simulink library "outp"  (Simulink 8.2)
settings: Solver=ode45  SolverMode=SingleTasking  StartTime=0.0  StopTime=10.0  RelTol=1e-3
undefined symbols (not defined in the file or in its folder): EPSILON, KOUTP_ACCSetSpeed_kph_defval, KOUTP_ACCSetSpeed_kph_maxval, KOUTP_ACCSetSpeed_kph_minval, KOUTP_ACCSetSpeed_kph_ovrdflg, KOUTP_ACCSetSpeed_kph_ovrdval, KOUTP_ACCSetSpeed_kph_srvcflg, KOUTP_ACCSetSpeed_kph_srvcval, KOUTP_ACCSetTimeGap_enum_defval, KOUTP_ACCSetTimeGap_enum_ovrdflg, KOUTP_ACCSetTimeGap_enum_ovrdval, KOUTP_ACCSetTimeGap_enum_srvcflg, KOUTP_ACCSetTimeGap_enum_srvcval, KOUTP_ACCSetTimeGapTmp_enum_defval, KOUTP_ACCSetTimeGapTmp_enum_ovrdflg, KOUTP_ACCSetTimeGapTmp_enum_ovrdval, KOUTP_ACCSetTimeGapTmp_enum_srvcflg, KOUTP_ACCSetTimeGapTmp_enum_srvcval, KOUTP_ACCWarningReq_flg_defval, KOUTP_ACCWarningReq_flg_ovrdflg, KOUTP_ACCWarningReq_flg_ovrdval, KOUTP_ACCWarningReq_flg_srvcflg, KOUTP_ACCWarningReq_flg_srvcval, KOUTP_ADAS1RollCnt_cnt_defval, KOUTP_ADAS1RollCnt_cnt_ovrdflg, KOUTP_ADAS1RollCnt_cnt_ovrdval, KOUTP_ADAS1RollCnt_cnt_srvcflg, KOUTP_ADAS1RollCnt_cnt_srvcval, KOUTP_ADAS2RollCnt_cnt_defval, KOUTP_ADAS2RollCnt_cnt_ovrdflg, KOUTP_ADAS2RollCnt_cnt_ovrdval, KOUTP_ADAS2RollCnt_cnt_srvcflg, KOUTP_ADAS2RollCnt_cnt_srvcval, KOUTP_ADAS3RollCnt_cnt_defval, KOUTP_ADAS3RollCnt_cnt_ovrdflg, KOUTP_ADAS3RollCnt_cnt_ovrdval, KOUTP_ADAS3RollCnt_cnt_srvcflg, KOUTP_ADAS3RollCnt_cnt_srvcval, KOUTP_ADASACCStatus_enum_defval, KOUTP_ADASACCStatus_enum_ovrdflg, KOUTP_ADASACCStatus_enum_ovrdval, KOUTP_ADASACCStatus_enum_srvcflg, KOUTP_ADASACCStatus_enum_srvcval, KOUTP_ADASFaultMode_enum_defval, KOUTP_ADASFaultMode_enum_ovrdflg, KOUTP_ADASFaultMode_enum_ovrdval, KOUTP_ADASFaultMode_enum_srvcflg, KOUTP_ADASFaultMode_enum_srvcval, KOUTP_ADASFunOffSoundReq_flg_defval, KOUTP_ADASFunOffSoundReq_flg_ovrdflg, KOUTP_ADASFunOffSoundReq_flg_ovrdval, KOUTP_ADASFunOffSoundReq_flg_srvcflg, KOUTP_ADASFunOffSoundReq_flg_srvcval, KOUTP_ADASFunOnSoundReq_flg_defval, KOUTP_ADASFunOnSoundReq_flg_ovrdflg, KOUTP_ADASFunOnSoundReq_flg_ovrdval, KOUTP_ADASFunOnSoundReq_flg_srvcflg, KOUTP_ADASFunOnSoundReq_flg_srvcval, KOUTP_ADASLFCStatus_enum_defval, KOUTP_ADASLFCStatus_enum_ovrdflg ... (+216)
libraries: outp x52, hcu_lib x8, simulink x3
(part 2 of 2)

== system outp/OUTP/OUTP/ADASFunOffSoundReq ==
  in : Inport
  use_default : Inport  Port=2
  KOUTP_LKAHMIStatus_enum_defval_C : Constant  Value=KOUTP_ADASFunOffSoundReq_flg_defval
  KOUTP_LKAHMIStatus_enum_ovrdflg_C : Constant  Value=KOUTP_ADASFunOffSoundReq_flg_ovrdflg
  KOUTP_LKAHMIStatus_enum_ovrdval_C : Constant  Value=KOUTP_ADASFunOffSoundReq_flg_ovrdval
  KOUTP_LKAHMIStatus_enum_srvcflg_C : Constant  Value=KOUTP_ADASFunOffSoundReq_flg_srvcflg
  KOUTP_LKAHMIStatus_enum_srvcval_C : Constant  Value=KOUTP_ADASFunOffSoundReq_flg_srvcval
  Switch1 : Switch  Criteria=u2 ~= 0  Threshold=0.5
  signal_out : outp/signal_out
  out : Outport
  wires:
  in/1 -> signal_out/1
  signal_out/1 -> Switch1/3
  use_default/1 -> Switch1/2
  Switch1/1 -> out/1
  KOUTP_LKAHMIStatus_enum_srvcflg_C/1 -> signal_out/2
  KOUTP_LKAHMIStatus_enum_srvcval_C/1 -> signal_out/3
  KOUTP_LKAHMIStatus_enum_ovrdflg_C/1 -> signal_out/4
  KOUTP_LKAHMIStatus_enum_ovrdval_C/1 -> signal_out/5
  KOUTP_LKAHMIStatus_enum_defval_C/1 -> Switch1/1

== system outp/OUTP/OUTP/ADASFunOnSoundReq ==
  in : Inport
  use_default : Inport  Port=2
  KOUTP_LKAHMIStatus_enum_defval_C : Constant  Value=KOUTP_ADASFunOnSoundReq_flg_defval
  KOUTP_LKAHMIStatus_enum_ovrdflg_C : Constant  Value=KOUTP_ADASFunOnSoundReq_flg_ovrdflg
  KOUTP_LKAHMIStatus_enum_ovrdval_C : Constant  Value=KOUTP_ADASFunOnSoundReq_flg_ovrdval
  KOUTP_LKAHMIStatus_enum_srvcflg_C : Constant  Value=KOUTP_ADASFunOnSoundReq_flg_srvcflg
  KOUTP_LKAHMIStatus_enum_srvcval_C : Constant  Value=KOUTP_ADASFunOnSoundReq_flg_srvcval
  Switch1 : Switch  Criteria=u2 ~= 0  Threshold=0.5
  signal_out : outp/signal_out
  out : Outport
  wires:
  KOUTP_LKAHMIStatus_enum_defval_C/1 -> Switch1/1
  KOUTP_LKAHMIStatus_enum_ovrdval_C/1 -> signal_out/5
  KOUTP_LKAHMIStatus_enum_ovrdflg_C/1 -> signal_out/4
  KOUTP_LKAHMIStatus_enum_srvcval_C/1 -> signal_out/3
  KOUTP_LKAHMIStatus_enum_srvcflg_C/1 -> signal_out/2
  Switch1/1 -> out/1
  use_default/1 -> Switch1/2
  signal_out/1 -> Switch1/3
  in/1 -> signal_out/1

== system outp/OUTP/OUTP/ADASLFCStatus ==
  in : Inport
  use_default : Inport  Port=2
  KOUTP_ADASLFCStatus_enum_defval_C : Constant  Value=KOUTP_ADASLFCStatus_enum_defval
  KOUTP_ADASLFCStatus_enum_ovrdflg_C : Constant  Value=KOUTP_ADASLFCStatus_enum_ovrdflg
  KOUTP_ADASLFCStatus_enum_ovrdval_C : Constant  Value=KOUTP_ADASLFCStatus_enum_ovrdval
  KOUTP_ADASLFCStatus_enum_srvcflg_C : Constant  Value=KOUTP_ADASLFCStatus_enum_srvcflg
  KOUTP_ADASLFCStatus_enum_srvcval_C : Constant  Value=KOUTP_ADASLFCStatus_enum_srvcval
  Switch1 : Switch  Criteria=u2 ~= 0  Threshold=0.5
  signal_out : outp/signal_out
  out : Outport
  wires:
  KOUTP_ADASLFCStatus_enum_defval_C/1 -> Switch1/1
  KOUTP_ADASLFCStatus_enum_ovrdval_C/1 -> signal_out/5
  KOUTP_ADASLFCStatus_enum_ovrdflg_C/1 -> signal_out/4
  KOUTP_ADASLFCStatus_enum_srvcval_C/1 -> signal_out/3
  KOUTP_ADASLFCStatus_enum_srvcflg_C/1 -> signal_out/2
  Switch1/1 -> out/1
  use_default/1 -> Switch1/2
  signal_out/1 -> Switch1/3
  in/1 -> signal_out/1

== system outp/OUTP/OUTP/ADASLKAStatus ==
  in : Inport
  use_default : Inport  Port=2
  KOUTP_ADASLKAStatus_enum_defval_C : Constant  Value=KOUTP_ADASLKAStatus_enum_defval
  KOUTP_ADASLKAStatus_enum_ovrdflg_C : Constant  Value=KOUTP_ADASLKAStatus_enum_ovrdflg
  KOUTP_ADASLKAStatus_enum_ovrdval_C : Constant  Value=KOUTP_ADASLKAStatus_enum_ovrdval
  KOUTP_ADASLKAStatus_enum_srvcflg_C : Constant  Value=KOUTP_ADASLKAStatus_enum_srvcflg
  KOUTP_ADASLKAStatus_enum_srvcval_C : Constant  Value=KOUTP_ADASLKAStatus_enum_srvcval
  Switch1 : Switch  Criteria=u2 ~= 0  Threshold=0.5
  signal_out : outp/signal_out
  out : Outport
  wires:
  in/1 -> signal_out/1
  signal_out/1 -> Switch1/3
  use_default/1 -> Switch1/2
  Switch1/1 -> out/1
  KOUTP_ADASLKAStatus_enum_srvcflg_C/1 -> signal_out/2
  KOUTP_ADASLKAStatus_enum_srvcval_C/1 -> signal_out/3
  KOUTP_ADASLKAStatus_enum_ovrdflg_C/1 -> signal_out/4
  KOUTP_ADASLKAStatus_enum_ovrdval_C/1 -> signal_out/5
  KOUTP_ADASLKAStatus_enum_defval_C/1 -> Switch1/1

== system outp/OUTP/OUTP/ADASMILReq ==
  in : Inport
  use_default : Inport  Port=2
  KOUTP_ADASMILReq_flg_defval_C : Constant  Value=KOUTP_ADASMILReq_flg_defval
  KOUTP_ADASMILReq_flg_ovrdflg_C : Constant  Value=KOUTP_ADASMILReq_flg_ovrdflg
  KOUTP_ADASMILReq_flg_ovrdval_C : Constant  Value=KOUTP_ADASMILReq_flg_ovrdval
  KOUTP_ADASMILReq_flg_srvcflg_C : Constant  Value=KOUTP_ADASMILReq_flg_srvcflg
  KOUTP_ADASMILReq_flg_srvcval_C : Constant  Value=KOUTP_ADASMILReq_flg_srvcval
  Switch1 : Switch  Criteria=u2 ~= 0  Threshold=0.5
  signal_out : outp/signal_out
  out : Outport
  wires:
  KOUTP_ADASMILReq_flg_defval_C/1 -> Switch1/1
  KOUTP_ADASMILReq_flg_ovrdval_C/1 -> signal_out/5
  KOUTP_ADASMILReq_flg_ovrdflg_C/1 -> signal_out/4
  KOUTP_ADASMILReq_flg_srvcval_C/1 -> signal_out/3
  KOUTP_ADASMILReq_flg_srvcflg_C/1 -> signal_out/2
  Switch1/1 -> out/1
  use_default/1 -> Switch1/2
  signal_out/1 -> Switch1/3
  in/1 -> signal_out/1

== system outp/OUTP/OUTP/AEBReq ==
  in : Inport
  use_default : Inport  Port=2
  KOUTP_AEBReq_flg_defval_C : Constant  Value=KOUTP_AEBReq_flg_defval
  KOUTP_AEBReq_flg_ovrdflg_C : Constant  Value=KOUTP_AEBReq_flg_ovrdflg
  KOUTP_AEBReq_flg_ovrdval_C : Constant  Value=KOUTP_AEBReq_flg_ovrdval
  KOUTP_AEBReq_flg_srvcflg_C : Constant  Value=KOUTP_AEBReq_flg_srvcflg
  KOUTP_AEBReq_flg_srvcval_C : Constant  Value=KOUTP_AEBReq_flg_srvcval
  Switch1 : Switch  Criteria=u2 ~= 0  Threshold=0.5
  signal_out : outp/signal_out
  out : Outport
  wires:
  in/1 -> signal_out/1
  signal_out/1 -> Switch1/3
  use_default/1 -> Switch1/2
  Switch1/1 -> out/1
  KOUTP_AEBReq_flg_srvcflg_C/1 -> signal_out/2
  KOUTP_AEBReq_flg_srvcval_C/1 -> signal_out/3
  KOUTP_AEBReq_flg_ovrdflg_C/1 -> signal_out/4
  KOUTP_AEBReq_flg_ovrdval_C/1 -> signal_out/5
  KOUTP_AEBReq_flg_defval_C/1 -> Switch1/1

== system outp/OUTP/OUTP/AEBReqAppl ==
  in : Inport
  use_default : Inport  Port=2
  KOUTP_AEBReqAppl_flg_defval_C : Constant  Value=KOUTP_AEBReqAppl_flg_defval
  KOUTP_AEBReqAppl_flg_ovrdflg_C : Constant  Value=KOUTP_AEBReqAppl_flg_ovrdflg
  KOUTP_AEBReqAppl_flg_ovrdval_C : Constant  Value=KOUTP_AEBReqAppl_flg_ovrdval
  KOUTP_AEBReqAppl_flg_srvcflg_C : Constant  Value=KOUTP_AEBReqAppl_flg_srvcflg
  KOUTP_AEBReqAppl_flg_srvcval_C : Constant  Value=KOUTP_AEBReqAppl_flg_srvcval
  Switch1 : Switch  Criteria=u2 ~= 0  Threshold=0.5
  signal_out : outp/signal_out
  out : Outport
  wires:
  KOUTP_AEBReqAppl_flg_defval_C/1 -> Switch1/1
  KOUTP_AEBReqAppl_flg_ovrdval_C/1 -> signal_out/5
  KOUTP_AEBReqAppl_flg_ovrdflg_C/1 -> signal_out/4
  KOUTP_AEBReqAppl_flg_srvcval_C/1 -> signal_out/3
  KOUTP_AEBReqAppl_flg_srvcflg_C/1 -> signal_out/2
  Switch1/1 -> out/1
  use_default/1 -> Switch1/2
  signal_out/1 -> Switch1/3
  in/1 -> signal_out/1

== system outp/OUTP/OUTP/AEBWarningReq ==
  in : Inport
  use_default : Inport  Port=2
  KOUTP_AEBWarningReq_flg_defval_C : Constant  Value=KOUTP_AEBWarningReq_flg_defval
  KOUTP_AEBWarningReq_flg_ovrdflg_C : Constant  Value=KOUTP_AEBWarningReq_flg_ovrdflg
  KOUTP_AEBWarningReq_flg_ovrdval_C : Constant  Value=KOUTP_AEBWarningReq_flg_ovrdval
  KOUTP_AEBWarningReq_flg_srvcflg_C : Constant  Value=KOUTP_AEBWarningReq_flg_srvcflg
  KOUTP_AEBWarningReq_flg_srvcval_C : Constant  Value=KOUTP_AEBWarningReq_flg_srvcval
  Switch1 : Switch  Criteria=u2 ~= 0  Threshold=0.5
  signal_out : outp/signal_out
  out : Outport
  wires:
  KOUTP_AEBWarningReq_flg_defval_C/1 -> Switch1/1
  KOUTP_AEBWarningReq_flg_ovrdval_C/1 -> signal_out/5
  KOUTP_AEBWarningReq_flg_ovrdflg_C/1 -> signal_out/4
  KOUTP_AEBWarningReq_flg_srvcval_C/1 -> signal_out/3
  KOUTP_AEBWarningReq_flg_srvcflg_C/1 -> signal_out/2
  Switch1/1 -> out/1
  use_default/1 -> Switch1/2
  signal_out/1 -> Switch1/3
  in/1 -> signal_out/1

== system outp/OUTP/OUTP/BrakeHapticReq ==
  in : Inport
  use_default : Inport  Port=2
  KOUTP_BrakeHapticReq_flg_defval_C : Constant  Value=KOUTP_BrakeHapticReq_flg_defval
  KOUTP_BrakeHapticReq_flg_ovrdflg_C : Constant  Value=KOUTP_BrakeHapticReq_flg_ovrdflg
  KOUTP_BrakeHapticReq_flg_ovrdval_C : Constant  Value=KOUTP_BrakeHapticReq_flg_ovrdval
  KOUTP_BrakeHapticReq_flg_srvcflg_C : Constant  Value=KOUTP_BrakeHapticReq_flg_srvcflg
  KOUTP_BrakeHapticReq_flg_srvcval_C : Constant  Value=KOUTP_BrakeHapticReq_flg_srvcval
  Switch1 : Switch  Criteria=u2 ~= 0  Threshold=0.5
  signal_out : outp/signal_out
  out : Outport
  wires:
  KOUTP_BrakeHapticReq_flg_defval_C/1 -> Switch1/1
  KOUTP_BrakeHapticReq_flg_ovrdval_C/1 -> signal_out/5
  KOUTP_BrakeHapticReq_flg_ovrdflg_C/1 -> signal_out/4
  KOUTP_BrakeHapticReq_flg_srvcval_C/1 -> signal_out/3
  KOUTP_BrakeHapticReq_flg_srvcflg_C/1 -> signal_out/2
  Switch1/1 -> out/1
  use_default/1 -> Switch1/2
  signal_out/1 -> Switch1/3
  in/1 -> signal_out/1

== system outp/OUTP/OUTP/BrakePrefillReq ==
  in : Inport
  use_default : Inport  Port=2
  KOUTP_BrakePrefillReq_flg_defval_C : Constant  Value=KOUTP_BrakePrefillReq_flg_defval
  KOUTP_BrakePrefillReq_flg_ovrdflg_C : Constant  Value=KOUTP_BrakePrefillReq_flg_ovrdflg
  KOUTP_BrakePrefillReq_flg_ovrdval_C : Constant  Value=KOUTP_BrakePrefillReq_flg_ovrdval
  KOUTP_BrakePrefillReq_flg_srvcflg_C : Constant  Value=KOUTP_BrakePrefillReq_flg_srvcflg
  KOUTP_BrakePrefillReq_flg_srvcval_C : Constant  Value=KOUTP_BrakePrefillReq_flg_srvcval
  Switch1 : Switch  Criteria=u2 ~= 0  Threshold=0.5
  signal_out : outp/signal_out
  out : Outport
  wires:
  in/1 -> signal_out/1
  signal_out/1 -> Switch1/3
  use_default/1 -> Switch1/2
  Switch1/1 -> out/1
  KOUTP_BrakePrefillReq_flg_srvcflg_C/1 -> signal_out/2
  KOUTP_BrakePrefillReq_flg_srvcval_C/1 -> signal_out/3
  KOUTP_BrakePrefillReq_flg_ovrdflg_C/1 -> signal_out/4
  KOUTP_BrakePrefillReq_flg_ovrdval_C/1 -> signal_out/5
  KOUTP_BrakePrefillReq_flg_defval_C/1 -> Switch1/1

== system outp/OUTP/OUTP/BrakePrefillReqAppl ==
  in : Inport
  use_default : Inport  Port=2
  KOUTP_BrakePrefillReqAppl_flg_defval_C : Constant  Value=KOUTP_BrakePrefillReqAppl_flg_defval
  KOUTP_BrakePrefillReqAppl_flg_ovrdflg_C : Constant  Value=KOUTP_BrakePrefillReqAppl_flg_ovrdflg
  KOUTP_BrakePrefillReqAppl_flg_ovrdval_C : Constant  Value=KOUTP_BrakePrefillReqAppl_flg_ovrdval
  KOUTP_BrakePrefillReqAppl_flg_srvcflg_C : Constant  Value=KOUTP_BrakePrefillReqAppl_flg_srvcflg
  KOUTP_BrakePrefillReqAppl_flg_srvcval_C : Constant  Value=KOUTP_BrakePrefillReqAppl_flg_srvcval
  Switch1 : Switch  Criteria=u2 ~= 0  Threshold=0.5
  signal_out : outp/signal_out
  out : Outport
  wires:
  KOUTP_BrakePrefillReqAppl_flg_defval_C/1 -> Switch1/1
  KOUTP_BrakePrefillReqAppl_flg_ovrdval_C/1 -> signal_out/5
  KOUTP_BrakePrefillReqAppl_flg_ovrdflg_C/1 -> signal_out/4
  KOUTP_BrakePrefillReqAppl_flg_srvcval_C/1 -> signal_out/3
  KOUTP_BrakePrefillReqAppl_flg_srvcflg_C/1 -> signal_out/2
  Switch1/1 -> out/1
  use_default/1 -> Switch1/2
  signal_out/1 -> Switch1/3
  in/1 -> signal_out/1

== system outp/OUTP/OUTP/DecReq ==
  in : Inport
  use_default : Inport  Port=2
  KOUTP_DecReq_mps2_defval_C : Constant  Value=KOUTP_DecReq_mps2_defval
  KOUTP_DecReq_mps2_ovrdflg_C : Constant  Value=KOUTP_DecReq_mps2_ovrdflg
  KOUTP_DecReq_mps2_ovrdval_C : Constant  Value=KOUTP_DecReq_mps2_ovrdval
  KOUTP_DecReq_mps2_srvcflg_C : Constant  Value=KOUTP_DecReq_mps2_srvcflg
  KOUTP_DecReq_mps2_srvcval_C : Constant  Value=KOUTP_DecReq_mps2_srvcval
  Switch1 : Switch  Criteria=u2 ~= 0  Threshold=0.5
  signal_out : outp/signal_out
  out : Outport
  wires:
  in/1 -> signal_out/1
  signal_out/1 -> Switch1/3
  use_default/1 -> Switch1/2
  Switch1/1 -> out/1
  KOUTP_DecReq_mps2_srvcflg_C/1 -> signal_out/2
  KOUTP_DecReq_mps2_srvcval_C/1 -> signal_out/3
  KOUTP_DecReq_mps2_ovrdflg_C/1 -> signal_out/4
  KOUTP_DecReq_mps2_ovrdval_C/1 -> signal_out/5
  KOUTP_DecReq_mps2_defval_C/1 -> Switch1/1

== system outp/OUTP/OUTP/DecReqAppl ==
  in : Inport
  use_default : Inport  Port=2
  KOUTP_DecReqAppl_flg_defval_C : Constant  Value=KOUTP_DecReqAppl_flg_defval
  KOUTP_DecReqAppl_flg_ovrdflg_C : Constant  Value=KOUTP_DecReqAppl_flg_ovrdflg
  KOUTP_DecReqAppl_flg_ovrdval_C : Constant  Value=KOUTP_DecReqAppl_flg_ovrdval
  KOUTP_DecReqAppl_flg_srvcflg_C : Constant  Value=KOUTP_DecReqAppl_flg_srvcflg
  KOUTP_DecReqAppl_flg_srvcval_C : Constant  Value=KOUTP_DecReqAppl_flg_srvcval
  Switch1 : Switch  Criteria=u2 ~= 0  Threshold=0.5
  signal_out : outp/signal_out
  out : Outport
  wires:
  KOUTP_DecReqAppl_flg_defval_C/1 -> Switch1/1
  KOUTP_DecReqAppl_flg_ovrdval_C/1 -> signal_out/5
  KOUTP_DecReqAppl_flg_ovrdflg_C/1 -> signal_out/4
  KOUTP_DecReqAppl_flg_srvcval_C/1 -> signal_out/3
  KOUTP_DecReqAppl_flg_srvcflg_C/1 -> signal_out/2
  Switch1/1 -> out/1
  use_default/1 -> Switch1/2
  signal_out/1 -> Switch1/3
  in/1 -> signal_out/1

== system outp/OUTP/OUTP/EPSModeReq ==
  in : Inport
  use_default : Inport  Port=2
  KOUTP_EPSModeReq_enum_defval_C : Constant  Value=KOUTP_EPSModeReq_enum_defval
  KOUTP_EPSModeReq_enum_ovrdflg_C : Constant  Value=KOUTP_EPSModeReq_enum_ovrdflg
  KOUTP_EPSModeReq_enum_ovrdval_C : Constant  Value=KOUTP_EPSModeReq_enum_ovrdval
  KOUTP_EPSModeReq_enum_srvcflg_C : Constant  Value=KOUTP_EPSModeReq_enum_srvcflg
  KOUTP_EPSModeReq_enum_srvcval_C : Constant  Value=KOUTP_EPSModeReq_enum_srvcval
  Switch1 : Switch  Criteria=u2 ~= 0  Threshold=0.5
  signal_out : outp/signal_out
  out : Outport
  wires:
  KOUTP_EPSModeReq_enum_defval_C/1 -> Switch1/1
  KOUTP_EPSModeReq_enum_ovrdval_C/1 -> signal_out/5
  KOUTP_EPSModeReq_enum_ovrdflg_C/1 -> signal_out/4
  KOUTP_EPSModeReq_enum_srvcval_C/1 -> signal_out/3
  KOUTP_EPSModeReq_enum_srvcflg_C/1 -> signal_out/2
  Switch1/1 -> out/1
  use_default/1 -> Switch1/2
  signal_out/1 -> Switch1/3
  in/1 -> signal_out/1

== system outp/OUTP/OUTP/FCWWarningReq ==
  in : Inport
  use_default : Inport  Port=2
  KOUTP_FCWWarningReq_flg_defval_C : Constant  Value=KOUTP_FCWWarningReq_flg_defval
  KOUTP_FCWWarningReq_flg_ovrdflg_C : Constant  Value=KOUTP_FCWWarningReq_flg_ovrdflg
  KOUTP_FCWWarningReq_flg_ovrdval_C : Constant  Value=KOUTP_FCWWarningReq_flg_ovrdval
  KOUTP_FCWWarningReq_flg_srvcflg_C : Constant  Value=KOUTP_FCWWarningReq_flg_srvcflg
  KOUTP_FCWWarningReq_flg_srvcval_C : Constant  Value=KOUTP_FCWWarningReq_flg_srvcval
  Switch1 : Switch  Criteria=u2 ~= 0  Threshold=0.5
  signal_out : outp/signal_out
  out : Outport
  wires:
  KOUTP_FCWWarningReq_flg_defval_C/1 -> Switch1/1
  KOUTP_FCWWarningReq_flg_ovrdval_C/1 -> signal_out/5
  KOUTP_FCWWarningReq_flg_ovrdflg_C/1 -> signal_out/4
  KOUTP_FCWWarningReq_flg_srvcval_C/1 -> signal_out/3
  KOUTP_FCWWarningReq_flg_srvcflg_C/1 -> signal_out/2
  Switch1/1 -> out/1
  use_default/1 -> Switch1/2
  signal_out/1 -> Switch1/3
  in/1 -> signal_out/1

== system outp/OUTP/OUTP/FaultWarningReq ==
  in : Inport
  use_default : Inport  Port=2
  KOUTP_FaultWarningReq_flg_defval_C : Constant  Value=KOUTP_FaultWarningReq_flg_defval
  KOUTP_FaultWarningReq_flg_ovrdflg_C : Constant  Value=KOUTP_FaultWarningReq_flg_ovrdflg
  KOUTP_FaultWarningReq_flg_ovrdval_C : Constant  Value=KOUTP_FaultWarningReq_flg_ovrdval
  KOUTP_FaultWarningReq_flg_srvcflg_C : Constant  Value=KOUTP_FaultWarningReq_flg_srvcflg
  KOUTP_FaultWarningReq_flg_srvcval_C : Constant  Value=KOUTP_FaultWarningReq_flg_srvcval
  Switch1 : Switch  Criteria=u2 ~= 0  Threshold=0.5
  signal_out : outp/signal_out
  out : Outport
  wires:
  KOUTP_FaultWarningReq_flg_defval_C/1 -> Switch1/1
  KOUTP_FaultWarningReq_flg_ovrdval_C/1 -> signal_out/5
  KOUTP_FaultWarningReq_flg_ovrdflg_C/1 -> signal_out/4
  KOUTP_FaultWarningReq_flg_srvcval_C/1 -> signal_out/3
  KOUTP_FaultWarningReq_flg_srvcflg_C/1 -> signal_out/2
  Switch1/1 -> out/1
  use_default/1 -> Switch1/2
  signal_out/1 -> Switch1/3
  in/1 -> signal_out/1

== system outp/OUTP/OUTP/ForceIdle ==
  in : Inport
  use_default : Inport  Port=2
  KOUTP_ForceIdle_flg_defval_C : Constant  Value=KOUTP_ForceIdle_flg_defval
  KOUTP_ForceIdle_flg_ovrdflg_C : Constant  Value=KOUTP_ForceIdle_flg_ovrdflg
  KOUTP_ForceIdle_flg_ovrdval_C : Constant  Value=KOUTP_ForceIdle_flg_ovrdval
  KOUTP_ForceIdle_flg_srvcflg_C : Constant  Value=KOUTP_ForceIdle_flg_srvcflg
  KOUTP_ForceIdle_flg_srvcval_C : Constant  Value=KOUTP_ForceIdle_flg_srvcval
  Switch1 : Switch  Criteria=u2 ~= 0  Threshold=0.5
  signal_out : outp/signal_out
  out : Outport
  wires:
  KOUTP_ForceIdle_flg_defval_C/1 -> Switch1/1
  KOUTP_ForceIdle_flg_ovrdval_C/1 -> signal_out/5
  KOUTP_ForceIdle_flg_ovrdflg_C/1 -> signal_out/4
  KOUTP_ForceIdle_flg_srvcval_C/1 -> signal_out/3
  KOUTP_ForceIdle_flg_srvcflg_C/1 -> signal_out/2
  Switch1/1 -> out/1
  use_default/1 -> Switch1/2
  signal_out/1 -> Switch1/3
  in/1 -> signal_out/1

== system outp/OUTP/OUTP/ForceIdleAppl ==
  in : Inport
  use_default : Inport  Port=2
  KOUTP_ForceIdleAppl_flg_defval_C : Constant  Value=KOUTP_ForceIdleAppl_flg_defval
  KOUTP_ForceIdleAppl_flg_ovrdflg_C : Constant  Value=KOUTP_ForceIdleAppl_flg_ovrdflg
  KOUTP_ForceIdleAppl_flg_ovrdval_C : Constant  Value=KOUTP_ForceIdleAppl_flg_ovrdval
  KOUTP_ForceIdleAppl_flg_srvcflg_C : Constant  Value=KOUTP_ForceIdleAppl_flg_srvcflg
  KOUTP_ForceIdleAppl_flg_srvcval_C : Constant  Value=KOUTP_ForceIdleAppl_flg_srvcval
  Switch1 : Switch  Criteria=u2 ~= 0  Threshold=0.5
  signal_out : outp/signal_out
  out : Outport
  wires:
  in/1 -> signal_out/1
  signal_out/1 -> Switch1/3
  use_default/1 -> Switch1/2
  Switch1/1 -> out/1
  KOUTP_ForceIdleAppl_flg_srvcflg_C/1 -> signal_out/2
  KOUTP_ForceIdleAppl_flg_srvcval_C/1 -> signal_out/3
  KOUTP_ForceIdleAppl_flg_ovrdflg_C/1 -> signal_out/4
  KOUTP_ForceIdleAppl_flg_ovrdval_C/1 -> signal_out/5
  KOUTP_ForceIdleAppl_flg_defval_C/1 -> Switch1/1

== system outp/OUTP/OUTP/ForceLowBeam ==
  in : Inport
  use_default : Inport  Port=2
  KOUTP_ADASMILReq_flg_defval_C : Constant  Value=KOUTP_ForceLowBeam_flg_defval
  KOUTP_ADASMILReq_flg_ovrdflg_C : Constant  Value=KOUTP_ForceLowBeam_flg_ovrdflg
  KOUTP_ADASMILReq_flg_ovrdval_C : Constant  Value=KOUTP_ForceLowBeam_flg_ovrdval
  KOUTP_ADASMILReq_flg_srvcflg_C : Constant  Value=KOUTP_ForceLowBeam_flg_srvcflg
  KOUTP_ADASMILReq_flg_srvcval_C : Constant  Value=KOUTP_ForceLowBeam_flg_srvcval
  Switch1 : Switch  Criteria=u2 ~= 0  Threshold=0.5
  signal_out : outp/signal_out
  out : Outport
  wires:
  in/1 -> signal_out/1
  signal_out/1 -> Switch1/3
  use_default/1 -> Switch1/2
  Switch1/1 -> out/1
  KOUTP_ADASMILReq_flg_srvcflg_C/1 -> signal_out/2
  KOUTP_ADASMILReq_flg_srvcval_C/1 -> signal_out/3
  KOUTP_ADASMILReq_flg_ovrdflg_C/1 -> signal_out/4
  KOUTP_ADASMILReq_flg_ovrdval_C/1 -> signal_out/5
  KOUTP_ADASMILReq_flg_defval_C/1 -> Switch1/1

== system outp/OUTP/OUTP/GearPosnReq ==
  in : Inport
  use_default : Inport  Port=2
  KOUTP_GearPosnReq_enum_defval_C : Constant  Value=KOUTP_GearPosnReq_enum_defval
  KOUTP_GearPosnReq_enum_ovrdflg_C : Constant  Value=KOUTP_GearPosnReq_enum_ovrdflg
  KOUTP_GearPosnReq_enum_ovrdval_C : Constant  Value=KOUTP_GearPosnReq_enum_ovrdval
  KOUTP_GearPosnReq_enum_srvcflg_C : Constant  Value=KOUTP_GearPosnReq_enum_srvcflg
  KOUTP_GearPosnReq_enum_srvcval_C : Constant  Value=KOUTP_GearPosnReq_enum_srvcval
  Switch1 : Switch  Criteria=u2 ~= 0  Threshold=0.5
  signal_out : outp/signal_out
  out : Outport
  wires:
  KOUTP_GearPosnReq_enum_defval_C/1 -> Switch1/1
  KOUTP_GearPosnReq_enum_ovrdval_C/1 -> signal_out/5
  KOUTP_GearPosnReq_enum_ovrdflg_C/1 -> signal_out/4
  KOUTP_GearPosnReq_enum_srvcval_C/1 -> signal_out/3
  KOUTP_GearPosnReq_enum_srvcflg_C/1 -> signal_out/2
  Switch1/1 -> out/1
  use_default/1 -> Switch1/2
  signal_out/1 -> Switch1/3
  in/1 -> signal_out/1

== system outp/OUTP/OUTP/GearPosnReqAppl ==
  in : Inport
  use_default : Inport  Port=2
  KOUTP_GearPosnReqAppl_flg_defval_C : Constant  Value=KOUTP_GearPosnReqAppl_flg_defval
  KOUTP_GearPosnReqAppl_flg_ovrdflg_C : Constant  Value=KOUTP_GearPosnReqAppl_flg_ovrdflg
  KOUTP_GearPosnReqAppl_flg_ovrdval_C : Constant  Value=KOUTP_GearPosnReqAppl_flg_ovrdval
  KOUTP_GearPosnReqAppl_flg_srvcflg_C : Constant  Value=KOUTP_GearPosnReqAppl_flg_srvcflg
  KOUTP_GearPosnReqAppl_flg_srvcval_C : Constant  Value=KOUTP_GearPosnReqAppl_flg_srvcval
  Switch1 : Switch  Criteria=u2 ~= 0  Threshold=0.5
  signal_out : outp/signal_out
  out : Outport
  wires:
  in/1 -> signal_out/1
  signal_out/1 -> Switch1/3
  use_default/1 -> Switch1/2
  Switch1/1 -> out/1
  KOUTP_GearPosnReqAppl_flg_srvcflg_C/1 -> signal_out/2
  KOUTP_GearPosnReqAppl_flg_srvcval_C/1 -> signal_out/3
  KOUTP_GearPosnReqAppl_flg_ovrdflg_C/1 -> signal_out/4
  KOUTP_GearPosnReqAppl_flg_ovrdval_C/1 -> signal_out/5
  KOUTP_GearPosnReqAppl_flg_defval_C/1 -> Switch1/1

== system outp/OUTP/OUTP/HazardWarningReq ==
  in : Inport
  use_default : Inport  Port=2
  KOUTP_HazardWarningReq_flg_defval_C : Constant  Value=KOUTP_HazardWarningReq_flg_defval
  KOUTP_HazardWarningReq_flg_ovrdflg_C : Constant  Value=KOUTP_HazardWarningReq_flg_ovrdflg
  KOUTP_HazardWarningReq_flg_ovrdval_C : Constant  Value=KOUTP_HazardWarningReq_flg_ovrdval
  KOUTP_HazardWarningReq_flg_srvcflg_C : Constant  Value=KOUTP_HazardWarningReq_flg_srvcflg
  KOUTP_HazardWarningReq_flg_srvcval_C : Constant  Value=KOUTP_HazardWarningReq_flg_srvcval
  Switch1 : Switch  Criteria=u2 ~= 0  Threshold=0.5
  signal_out : outp/signal_out
  out : Outport
  wires:
  in/1 -> signal_out/1
  signal_out/1 -> Switch1/3
  use_default/1 -> Switch1/2
  Switch1/1 -> out/1
  KOUTP_HazardWarningReq_flg_srvcflg_C/1 -> signal_out/2
  KOUTP_HazardWarningReq_flg_srvcval_C/1 -> signal_out/3
  KOUTP_HazardWarningReq_flg_ovrdflg_C/1 -> signal_out/4
  KOUTP_HazardWarningReq_flg_ovrdval_C/1 -> signal_out/5
  KOUTP_HazardWarningReq_flg_defval_C/1 -> Switch1/1

== system outp/OUTP/OUTP/IGSAWarningReq ==
  in : Inport
  use_default : Inport  Port=2
  KOUTP_IGSAWarningReq_flg_defval_C : Constant  Value=KOUTP_IGSAWarningReq_flg_defval
  KOUTP_IGSAWarningReq_flg_ovrdflg_C : Constant  Value=KOUTP_IGSAWarningReq_flg_ovrdflg
  KOUTP_IGSAWarningReq_flg_ovrdval_C : Constant  Value=KOUTP_IGSAWarningReq_flg_ovrdval
  KOUTP_IGSAWarningReq_flg_srvcflg_C : Constant  Value=KOUTP_IGSAWarningReq_flg_srvcflg
  KOUTP_IGSAWarningReq_flg_srvcval_C : Constant  Value=KOUTP_IGSAWarningReq_flg_srvcval
  Switch1 : Switch  Criteria=u2 ~= 0  Threshold=0.5
  signal_out : outp/signal_out
  out : Outport
  wires:
  in/1 -> signal_out/1
  signal_out/1 -> Switch1/3
  use_default/1 -> Switch1/2
  Switch1/1 -> out/1
  KOUTP_IGSAWarningReq_flg_srvcflg_C/1 -> signal_out/2
  KOUTP_IGSAWarningReq_flg_srvcval_C/1 -> signal_out/3
  KOUTP_IGSAWarningReq_flg_ovrdflg_C/1 -> signal_out/4
  KOUTP_IGSAWarningReq_flg_ovrdval_C/1 -> signal_out/5
  KOUTP_IGSAWarningReq_flg_defval_C/1 -> Switch1/1

== system outp/OUTP/OUTP/LFCHMIStatus ==
  in : Inport
  use_default : Inport  Port=2
  KOUTP_LFCHMIStatus_enum_defval_C : Constant  Value=KOUTP_LFCHMIStatus_enum_defval
  KOUTP_LFCHMIStatus_enum_ovrdflg_C : Constant  Value=KOUTP_LFCHMIStatus_enum_ovrdflg
  KOUTP_LFCHMIStatus_enum_ovrdval_C : Constant  Value=KOUTP_LFCHMIStatus_enum_ovrdval
  KOUTP_LFCHMIStatus_enum_srvcflg_C : Constant  Value=KOUTP_LFCHMIStatus_enum_srvcflg
  KOUTP_LFCHMIStatus_enum_srvcval_C : Constant  Value=KOUTP_LFCHMIStatus_enum_srvcval
  Switch1 : Switch  Criteria=u2 ~= 0  Threshold=0.5
  signal_out : outp/signal_out
  out : Outport
  wires:
  in/1 -> signal_out/1
  signal_out/1 -> Switch1/3
  use_default/1 -> Switch1/2
  Switch1/1 -> out/1
  KOUTP_LFCHMIStatus_enum_srvcflg_C/1 -> signal_out/2
  KOUTP_LFCHMIStatus_enum_srvcval_C/1 -> signal_out/3
  KOUTP_LFCHMIStatus_enum_ovrdflg_C/1 -> signal_out/4
  KOUTP_LFCHMIStatus_enum_ovrdval_C/1 -> signal_out/5
  KOUTP_LFCHMIStatus_enum_defval_C/1 -> Switch1/1

== system outp/OUTP/OUTP/LFCTransGain ==
  in : Inport
  use_default : Inport  Port=2
  KOUTP_LFCTransGain_rat_defval_C : Constant  Value=KOUTP_LFCTransGain_rat_defval
  KOUTP_LFCTransGain_rat_ovrdflg_C : Constant  Value=KOUTP_LFCTransGain_rat_ovrdflg
  KOUTP_LFCTransGain_rat_ovrdval_C : Constant  Value=KOUTP_LFCTransGain_rat_ovrdval
  KOUTP_LFCTransGain_rat_srvcflg_C : Constant  Value=KOUTP_LFCTransGain_rat_srvcflg
  KOUTP_LFCTransGain_rat_srvcval_C : Constant  Value=KOUTP_LFCTransGain_rat_srvcval
  Switch1 : Switch  Criteria=u2 ~= 0  Threshold=0.5
  signal_out : outp/signal_out
  out : Outport
  wires:
  in/1 -> signal_out/1
  signal_out/1 -> Switch1/3
  use_default/1 -> Switch1/2
  Switch1/1 -> out/1
  KOUTP_LFCTransGain_rat_srvcflg_C/1 -> signal_out/2
  KOUTP_LFCTransGain_rat_srvcval_C/1 -> signal_out/3
  KOUTP_LFCTransGain_rat_ovrdflg_C/1 -> signal_out/4
  KOUTP_LFCTransGain_rat_ovrdval_C/1 -> signal_out/5
  KOUTP_LFCTransGain_rat_defval_C/1 -> Switch1/1

== system outp/OUTP/OUTP/LFCTransGainAppl ==
  in : Inport
  use_default : Inport  Port=2
  KOUTP_LFCTransGainAppl_flg_defval_C : Constant  Value=KOUTP_LFCTransGainAppl_flg_defval
  KOUTP_LFCTransGainAppl_flg_ovrdflg_C : Constant  Value=KOUTP_LFCTransGainAppl_flg_ovrdflg
  KOUTP_LFCTransGainAppl_flg_ovrdval_C : Constant  Value=KOUTP_LFCTransGainAppl_flg_ovrdval
  KOUTP_LFCTransGainAppl_flg_srvcflg_C : Constant  Value=KOUTP_LFCTransGainAppl_flg_srvcflg
  KOUTP_LFCTransGainAppl_flg_srvcval_C : Constant  Value=KOUTP_LFCTransGainAppl_flg_srvcval
  Switch1 : Switch  Criteria=u2 ~= 0  Threshold=0.5
  signal_out : outp/signal_out
  out : Outport
  wires:
  in/1 -> signal_out/1
  signal_out/1 -> Switch1/3
  use_default/1 -> Switch1/2
  Switch1/1 -> out/1
  KOUTP_LFCTransGainAppl_flg_srvcflg_C/1 -> signal_out/2
  KOUTP_LFCTransGainAppl_flg_srvcval_C/1 -> signal_out/3
  KOUTP_LFCTransGainAppl_flg_ovrdflg_C/1 -> signal_out/4
  KOUTP_LFCTransGainAppl_flg_ovrdval_C/1 -> signal_out/5
  KOUTP_LFCTransGainAppl_flg_defval_C/1 -> Switch1/1

== system outp/OUTP/OUTP/LFCWarningReq ==
  in : Inport
  use_default : Inport  Port=2
  KOUTP_LKAHMIStatus_enum_defval_C : Constant  Value=KOUTP_LFCWarningReq_flg_defval
  KOUTP_LKAHMIStatus_enum_ovrdflg_C : Constant  Value=KOUTP_LFCWarningReq_flg_ovrdflg
  KOUTP_LKAHMIStatus_enum_ovrdval_C : Constant  Value=KOUTP_LFCWarningReq_flg_ovrdval
  KOUTP_LKAHMIStatus_enum_srvcflg_C : Constant  Value=KOUTP_LFCWarningReq_flg_srvcflg
  KOUTP_LKAHMIStatus_enum_srvcval_C : Constant  Value=KOUTP_LFCWarningReq_flg_srvcval
  Switch1 : Switch  Criteria=u2 ~= 0  Threshold=0.5
  signal_out : outp/signal_out
  out : Outport
  wires:
  in/1 -> signal_out/1
  signal_out/1 -> Switch1/3
  use_default/1 -> Switch1/2
  Switch1/1 -> out/1
  KOUTP_LKAHMIStatus_enum_srvcflg_C/1 -> signal_out/2
  KOUTP_LKAHMIStatus_enum_srvcval_C/1 -> signal_out/3
  KOUTP_LKAHMIStatus_enum_ovrdflg_C/1 -> signal_out/4
  KOUTP_LKAHMIStatus_enum_ovrdval_C/1 -> signal_out/5
  KOUTP_LKAHMIStatus_enum_defval_C/1 -> Switch1/1

== system outp/OUTP/OUTP/LKAHMIStatus ==
  in : Inport
  use_default : Inport  Port=2
  KOUTP_LKAHMIStatus_enum_defval_C : Constant  Value=KOUTP_LKAHMIStatus_enum_defval
  KOUTP_LKAHMIStatus_enum_ovrdflg_C : Constant  Value=KOUTP_LKAHMIStatus_enum_ovrdflg
  KOUTP_LKAHMIStatus_enum_ovrdval_C : Constant  Value=KOUTP_LKAHMIStatus_enum_ovrdval
  KOUTP_LKAHMIStatus_enum_srvcflg_C : Constant  Value=KOUTP_LKAHMIStatus_enum_srvcflg
  KOUTP_LKAHMIStatus_enum_srvcval_C : Constant  Value=KOUTP_LKAHMIStatus_enum_srvcval
  Switch1 : Switch  Criteria=u2 ~= 0  Threshold=0.5
  signal_out : outp/signal_out
  out : Outport
  wires:
  KOUTP_LKAHMIStatus_enum_defval_C/1 -> Switch1/1
  KOUTP_LKAHMIStatus_enum_ovrdval_C/1 -> signal_out/5
  KOUTP_LKAHMIStatus_enum_ovrdflg_C/1 -> signal_out/4
  KOUTP_LKAHMIStatus_enum_srvcval_C/1 -> signal_out/3
  KOUTP_LKAHMIStatus_enum_srvcflg_C/1 -> signal_out/2
  Switch1/1 -> out/1
  use_default/1 -> Switch1/2
  signal_out/1 -> Switch1/3
  in/1 -> signal_out/1

== system outp/OUTP/OUTP/LeftLaneLampMode ==
  in : Inport
  use_default : Inport  Port=2
  KOUTP_LeftLaneLampMode_enum_defval_C : Constant  Value=KOUTP_LeftLaneLampMode_enum_defval
  KOUTP_LeftLaneLampMode_enum_ovrdflg_C : Constant  Value=KOUTP_LeftLaneLampMode_enum_ovrdflg
  KOUTP_LeftLaneLampMode_enum_ovrdval_C : Constant  Value=KOUTP_LeftLaneLampMode_enum_ovrdval
  KOUTP_LeftLaneLampMode_enum_srvcflg_C : Constant  Value=KOUTP_LeftLaneLampMode_enum_srvcflg
  KOUTP_LeftLaneLampMode_enum_srvcval_C : Constant  Value=KOUTP_LeftLaneLampMode_enum_srvcval
  Switch1 : Switch  Criteria=u2 ~= 0  Threshold=0.5
  signal_out : outp/signal_out
  out : Outport
  wires:
  in/1 -> signal_out/1
  signal_out/1 -> Switch1/3
  use_default/1 -> Switch1/2
  Switch1/1 -> out/1
  KOUTP_LeftLaneLampMode_enum_srvcflg_C/1 -> signal_out/2
  KOUTP_LeftLaneLampMode_enum_srvcval_C/1 -> signal_out/3
  KOUTP_LeftLaneLampMode_enum_ovrdflg_C/1 -> signal_out/4
  KOUTP_LeftLaneLampMode_enum_ovrdval_C/1 -> signal_out/5
  KOUTP_LeftLaneLampMode_enum_defval_C/1 -> Switch1/1

== system outp/OUTP/OUTP/NumberOfTargets ==
  in : Inport
  use_default : Inport  Port=2
  KOUTP_LKAHMIStatus_enum_defval_C : Constant  Value=KOUTP_NumberOfTargets_num_defval
  KOUTP_LKAHMIStatus_enum_ovrdflg_C : Constant  Value=KOUTP_NumberOfTargets_num_ovrdflg
  KOUTP_LKAHMIStatus_enum_ovrdval_C : Constant  Value=KOUTP_NumberOfTargets_num_ovrdval
  KOUTP_LKAHMIStatus_enum_srvcflg_C : Constant  Value=KOUTP_NumberOfTargets_num_srvcflg
  KOUTP_LKAHMIStatus_enum_srvcval_C : Constant  Value=KOUTP_NumberOfTargets_num_srvcval
  Switch1 : Switch  Criteria=u2 ~= 0  Threshold=0.5
  signal_out : outp/signal_out
  out : Outport
  wires:
  in/1 -> signal_out/1
  signal_out/1 -> Switch1/3
  use_default/1 -> Switch1/2
  Switch1/1 -> out/1
  KOUTP_LKAHMIStatus_enum_srvcflg_C/1 -> signal_out/2
  KOUTP_LKAHMIStatus_enum_srvcval_C/1 -> signal_out/3
  KOUTP_LKAHMIStatus_enum_ovrdflg_C/1 -> signal_out/4
  KOUTP_LKAHMIStatus_enum_ovrdval_C/1 -> signal_out/5
  KOUTP_LKAHMIStatus_enum_defval_C/1 -> Switch1/1

== system outp/OUTP/OUTP/PTTqReq ==
  in : Inport
  use_default : Inport  Port=2
  KOUTP_PTTqReq_Nm_defval_C : Constant  Value=KOUTP_PTTqReq_Nm_defval
  KOUTP_PTTqReq_Nm_ovrdflg_C : Constant  Value=KOUTP_PTTqReq_Nm_ovrdflg
  KOUTP_PTTqReq_Nm_ovrdval_C : Constant  Value=KOUTP_PTTqReq_Nm_ovrdval
  KOUTP_PTTqReq_Nm_srvcflg_C : Constant  Value=KOUTP_PTTqReq_Nm_srvcflg
  KOUTP_PTTqReq_Nm_srvcval_C : Constant  Value=KOUTP_PTTqReq_Nm_srvcval
  Switch1 : Switch  Criteria=u2 ~= 0  Threshold=0.5
  signal_out : outp/signal_out
  out : Outport
  wires:
  KOUTP_PTTqReq_Nm_defval_C/1 -> Switch1/1
  KOUTP_PTTqReq_Nm_ovrdval_C/1 -> signal_out/5
  KOUTP_PTTqReq_Nm_ovrdflg_C/1 -> signal_out/4
  KOUTP_PTTqReq_Nm_srvcval_C/1 -> signal_out/3
  KOUTP_PTTqReq_Nm_srvcflg_C/1 -> signal_out/2
  Switch1/1 -> out/1
  use_default/1 -> Switch1/2
  signal_out/1 -> Switch1/3
  in/1 -> signal_out/1

== system outp/OUTP/OUTP/PTTqReqAppl ==
  in : Inport
  use_default : Inport  Port=2
  KOUTP_PTTqReqAppl_flg_defval_C : Constant  Value=KOUTP_PTTqReqAppl_flg_defval
  KOUTP_PTTqReqAppl_flg_ovrdflg_C : Constant  Value=KOUTP_PTTqReqAppl_flg_ovrdflg
  KOUTP_PTTqReqAppl_flg_ovrdval_C : Constant  Value=KOUTP_PTTqReqAppl_flg_ovrdval
  KOUTP_PTTqReqAppl_flg_srvcflg_C : Constant  Value=KOUTP_PTTqReqAppl_flg_srvcflg
  KOUTP_PTTqReqAppl_flg_srvcval_C : Constant  Value=KOUTP_PTTqReqAppl_flg_srvcval
  Switch1 : Switch  Criteria=u2 ~= 0  Threshold=0.5
  signal_out : outp/signal_out
  out : Outport
  wires:
  in/1 -> signal_out/1
  signal_out/1 -> Switch1/3
  use_default/1 -> Switch1/2
  Switch1/1 -> out/1
  KOUTP_PTTqReqAppl_flg_srvcflg_C/1 -> signal_out/2
  KOUTP_PTTqReqAppl_flg_srvcval_C/1 -> signal_out/3
  KOUTP_PTTqReqAppl_flg_ovrdflg_C/1 -> signal_out/4
  KOUTP_PTTqReqAppl_flg_ovrdval_C/1 -> signal_out/5
  KOUTP_PTTqReqAppl_flg_defval_C/1 -> Switch1/1

== system outp/OUTP/OUTP/RightLaneLampMode ==
  in : Inport
  use_default : Inport  Port=2
  KOUTP_RightLaneLampMode_enum_defval_C : Constant  Value=KOUTP_RightLaneLampMode_enum_defval
  KOUTP_RightLaneLampMode_enum_ovrdflg_C : Constant  Value=KOUTP_RightLaneLampMode_enum_ovrdflg
  KOUTP_RightLaneLampMode_enum_ovrdval_C : Constant  Value=KOUTP_RightLaneLampMode_enum_ovrdval
  KOUTP_RightLaneLampMode_enum_srvcflg_C : Constant  Value=KOUTP_RightLaneLampMode_enum_srvcflg
  KOUTP_RightLaneLampMode_enum_srvcval_C : Constant  Value=KOUTP_RightLaneLampMode_enum_srvcval
  Switch1 : Switch  Criteria=u2 ~= 0  Threshold=0.5
  signal_out : outp/signal_out
  out : Outport
  wires:
  KOUTP_RightLaneLampMode_enum_defval_C/1 -> Switch1/1
  KOUTP_RightLaneLampMode_enum_ovrdval_C/1 -> signal_out/5
  KOUTP_RightLaneLampMode_enum_ovrdflg_C/1 -> signal_out/4
  KOUTP_RightLaneLampMode_enum_srvcval_C/1 -> signal_out/3
  KOUTP_RightLaneLampMode_enum_srvcflg_C/1 -> signal_out/2
  Switch1/1 -> out/1
  use_default/1 -> Switch1/2
  signal_out/1 -> Switch1/3
  in/1 -> signal_out/1

== system outp/OUTP/OUTP/RollCnt ==
  max : Inport
  Trigger : TriggerPort  TriggerType=function-call  PortDimensions=1
  Add : Sum
  Constant : Constant  OutDataTypeStr=Inherit: Inherit via back propagation
  Constant1 : Constant  Value=0  OutDataTypeStr=Inherit: Inherit via back propagation
  Data Type Conversion6 : DataTypeConversion  OutDataTypeStr=uint8
  Relational Operator : RelationalOperator  Operator=>  OutDataTypeStr=boolean
  Switch2 : Switch  Criteria=u2 ~= 0
  Unit Delay1 : UnitDelay  SampleTime=-1
  out : Outport
  wires:
  Constant/1 -> Add/1
  Add/1 -> Switch2/3, Relational Operator/1
  Unit Delay1/1 -> Add/2
  Constant1/1 -> Switch2/1
  Switch2/1 -> Unit Delay1/1, Data Type Conversion6/1
  max/1 -> Relational Operator/2
  Relational Operator/1 -> Switch2/2
  Data Type Conversion6/1 -> out/1

== system outp/OUTP/OUTP/RollCnt1 ==
  max : Inport
  Trigger : TriggerPort  TriggerType=function-call  PortDimensions=1
  Add : Sum
  Constant : Constant  OutDataTypeStr=Inherit: Inherit via back propagation
  Constant1 : Constant  Value=0  OutDataTypeStr=Inherit: Inherit via back propagation
  Data Type Conversion6 : DataTypeConversion  OutDataTypeStr=uint8
  Relational Operator : RelationalOperator  Operator=>  OutDataTypeStr=boolean
  Switch2 : Switch  Criteria=u2 ~= 0
  Unit Delay1 : UnitDelay  SampleTime=-1
  out : Outport
  wires:
  Data Type Conversion6/1 -> out/1
  Relational Operator/1 -> Switch2/2
  max/1 -> Relational Operator/2
  Switch2/1 -> Data Type Conversion6/1, Unit Delay1/1
  Constant1/1 -> Switch2/1
  Unit Delay1/1 -> Add/2
  Add/1 -> Relational Operator/1, Switch2/3
  Constant/1 -> Add/1

== system outp/OUTP/OUTP/RollCnt2 ==
  max : Inport
  Trigger : TriggerPort  TriggerType=function-call  PortDimensions=1
  Add : Sum
  Constant : Constant  OutDataTypeStr=Inherit: Inherit via back propagation
  Constant1 : Constant  Value=0  OutDataTypeStr=Inherit: Inherit via back propagation
  Data Type Conversion6 : DataTypeConversion  OutDataTypeStr=uint8
  Relational Operator : RelationalOperator  Operator=>  OutDataTypeStr=boolean
  Switch2 : Switch  Criteria=u2 ~= 0
  Unit Delay1 : UnitDelay  SampleTime=-1
  out : Outport
  wires:
  Constant/1 -> Add/1
  Add/1 -> Switch2/3, Relational Operator/1
  Unit Delay1/1 -> Add/2
  Constant1/1 -> Switch2/1
  Switch2/1 -> Unit Delay1/1, Data Type Conversion6/1
  max/1 -> Relational Operator/2
  Relational Operator/1 -> Switch2/2
  Data Type Conversion6/1 -> out/1

== system outp/OUTP/OUTP/ShiftPosnReq ==
  in : Inport
  use_default : Inport  Port=2
  KOUTP_ShiftPosnReq_enum_defval_C : Constant  Value=KOUTP_ShiftPosnReq_enum_defval
  KOUTP_ShiftPosnReq_enum_ovrdflg_C : Constant  Value=KOUTP_ShiftPosnReq_enum_ovrdflg
  KOUTP_ShiftPosnReq_enum_ovrdval_C : Constant  Value=KOUTP_ShiftPosnReq_enum_ovrdval
  KOUTP_ShiftPosnReq_enum_srvcflg_C : Constant  Value=KOUTP_ShiftPosnReq_enum_srvcflg
  KOUTP_ShiftPosnReq_enum_srvcval_C : Constant  Value=KOUTP_ShiftPosnReq_enum_srvcval
  Switch1 : Switch  Criteria=u2 ~= 0  Threshold=0.5
  signal_out : outp/signal_out
  out : Outport
  wires:
  KOUTP_ShiftPosnReq_enum_defval_C/1 -> Switch1/1
  KOUTP_ShiftPosnReq_enum_ovrdval_C/1 -> signal_out/5
  KOUTP_ShiftPosnReq_enum_ovrdflg_C/1 -> signal_out/4
  KOUTP_ShiftPosnReq_enum_srvcval_C/1 -> signal_out/3
  KOUTP_ShiftPosnReq_enum_srvcflg_C/1 -> signal_out/2
  Switch1/1 -> out/1
  use_default/1 -> Switch1/2
  signal_out/1 -> Switch1/3
  in/1 -> signal_out/1

== system outp/OUTP/OUTP/ShiftPosnReqAppl ==
  in : Inport
  use_default : Inport  Port=2
  KOUTP_ShiftPosnReqAppl_flg_defval_C : Constant  Value=KOUTP_ShiftPosnReqAppl_flg_defval
  KOUTP_ShiftPosnReqAppl_flg_ovrdflg_C : Constant  Value=KOUTP_ShiftPosnReqAppl_flg_ovrdflg
  KOUTP_ShiftPosnReqAppl_flg_ovrdval_C : Constant  Value=KOUTP_ShiftPosnReqAppl_flg_ovrdval
  KOUTP_ShiftPosnReqAppl_flg_srvcflg_C : Constant  Value=KOUTP_ShiftPosnReqAppl_flg_srvcflg
  KOUTP_ShiftPosnReqAppl_flg_srvcval_C : Constant  Value=KOUTP_ShiftPosnReqAppl_flg_srvcval
  Switch1 : Switch  Criteria=u2 ~= 0  Threshold=0.5
  signal_out : outp/signal_out
  out : Outport
  wires:
  in/1 -> signal_out/1
  signal_out/1 -> Switch1/3
  use_default/1 -> Switch1/2
  Switch1/1 -> out/1
  KOUTP_ShiftPosnReqAppl_flg_srvcflg_C/1 -> signal_out/2
  KOUTP_ShiftPosnReqAppl_flg_srvcval_C/1 -> signal_out/3
  KOUTP_ShiftPosnReqAppl_flg_ovrdflg_C/1 -> signal_out/4
  KOUTP_ShiftPosnReqAppl_flg_ovrdval_C/1 -> signal_out/5
  KOUTP_ShiftPosnReqAppl_flg_defval_C/1 -> Switch1/1

== system outp/OUTP/OUTP/StrAngAppl ==
  in : Inport
  use_default : Inport  Port=2
  KOUTP_StrAngAppl_flg_defval_C : Constant  Value=KOUTP_StrAngAppl_flg_defval
  KOUTP_StrAngAppl_flg_ovrdflg_C : Constant  Value=KOUTP_StrAngAppl_flg_ovrdflg
  KOUTP_StrAngAppl_flg_ovrdval_C : Constant  Value=KOUTP_StrAngAppl_flg_ovrdval
  KOUTP_StrAngAppl_flg_srvcflg_C : Constant  Value=KOUTP_StrAngAppl_flg_srvcflg
  KOUTP_StrAngAppl_flg_srvcval_C : Constant  Value=KOUTP_StrAngAppl_flg_srvcval
  Switch1 : Switch  Criteria=u2 ~= 0  Threshold=0.5
  signal_out : outp/signal_out
  out : Outport
  wires:
  in/1 -> signal_out/1
  signal_out/1 -> Switch1/3
  use_default/1 -> Switch1/2
  Switch1/1 -> out/1
  KOUTP_StrAngAppl_flg_srvcflg_C/1 -> signal_out/2
  KOUTP_StrAngAppl_flg_srvcval_C/1 -> signal_out/3
  KOUTP_StrAngAppl_flg_ovrdflg_C/1 -> signal_out/4
  KOUTP_StrAngAppl_flg_ovrdval_C/1 -> signal_out/5
  KOUTP_StrAngAppl_flg_defval_C/1 -> Switch1/1

== system outp/OUTP/OUTP/StrAngReq ==
  in : Inport
  use_default : Inport  Port=2
  KOUTP_StrAngReq_deg_defval_C : Constant  Value=KOUTP_StrAngReq_deg_defval
  KOUTP_StrAngReq_deg_ovrdflg_C : Constant  Value=KOUTP_StrAngReq_deg_ovrdflg
  KOUTP_StrAngReq_deg_ovrdval_C : Constant  Value=KOUTP_StrAngReq_deg_ovrdval
  KOUTP_StrAngReq_deg_srvcflg_C : Constant  Value=KOUTP_StrAngReq_deg_srvcflg
  KOUTP_StrAngReq_deg_srvcval_C : Constant  Value=KOUTP_StrAngReq_deg_srvcval
  Switch1 : Switch  Criteria=u2 ~= 0  Threshold=0.5
  signal_out : outp/signal_out
  out : Outport
  wires:
  in/1 -> signal_out/1
  signal_out/1 -> Switch1/3
  use_default/1 -> Switch1/2
  Switch1/1 -> out/1
  KOUTP_StrAngReq_deg_srvcflg_C/1 -> signal_out/2
  KOUTP_StrAngReq_deg_srvcval_C/1 -> signal_out/3
  KOUTP_StrAngReq_deg_ovrdflg_C/1 -> signal_out/4
  KOUTP_StrAngReq_deg_ovrdval_C/1 -> signal_out/5
  KOUTP_StrAngReq_deg_defval_C/1 -> Switch1/1

== system outp/OUTP/OUTP/StrTqAppl ==
  in : Inport
  use_default : Inport  Port=2
  KOUTP_StrTqAppl_flg_defval_C : Constant  Value=KOUTP_StrTqAppl_flg_defval
  KOUTP_StrTqAppl_flg_ovrdflg_C : Constant  Value=KOUTP_StrTqAppl_flg_ovrdflg
  KOUTP_StrTqAppl_flg_ovrdval_C : Constant  Value=KOUTP_StrTqAppl_flg_ovrdval
  KOUTP_StrTqAppl_flg_srvcflg_C : Constant  Value=KOUTP_StrTqAppl_flg_srvcflg
  KOUTP_StrTqAppl_flg_srvcval_C : Constant  Value=KOUTP_StrTqAppl_flg_srvcval
  Switch1 : Switch  Criteria=u2 ~= 0  Threshold=0.5
  signal_out : outp/signal_out
  out : Outport
  wires:
  KOUTP_StrTqAppl_flg_defval_C/1 -> Switch1/1
  KOUTP_StrTqAppl_flg_ovrdval_C/1 -> signal_out/5
  KOUTP_StrTqAppl_flg_ovrdflg_C/1 -> signal_out/4
  KOUTP_StrTqAppl_flg_srvcval_C/1 -> signal_out/3
  KOUTP_StrTqAppl_flg_srvcflg_C/1 -> signal_out/2
  Switch1/1 -> out/1
  use_default/1 -> Switch1/2
  signal_out/1 -> Switch1/3
  in/1 -> signal_out/1

== system outp/OUTP/OUTP/StrTqReq ==
  in : Inport
  use_default : Inport  Port=2
  KOUTP_StrTqReq_Nm_defval_C : Constant  Value=KOUTP_StrTqReq_Nm_defval
  KOUTP_StrTqReq_Nm_ovrdflg_C : Constant  Value=KOUTP_StrTqReq_Nm_ovrdflg
  KOUTP_StrTqReq_Nm_ovrdval_C : Constant  Value=KOUTP_StrTqReq_Nm_ovrdval
  KOUTP_StrTqReq_Nm_srvcflg_C : Constant  Value=KOUTP_StrTqReq_Nm_srvcflg
  KOUTP_StrTqReq_Nm_srvcval_C : Constant  Value=KOUTP_StrTqReq_Nm_srvcval
  Switch1 : Switch  Criteria=u2 ~= 0  Threshold=0.5
  signal_out : outp/signal_out
  out : Outport
  wires:
  KOUTP_StrTqReq_Nm_defval_C/1 -> Switch1/1
  KOUTP_StrTqReq_Nm_ovrdval_C/1 -> signal_out/5
  KOUTP_StrTqReq_Nm_ovrdflg_C/1 -> signal_out/4
  KOUTP_StrTqReq_Nm_srvcval_C/1 -> signal_out/3
  KOUTP_StrTqReq_Nm_srvcflg_C/1 -> signal_out/2
  Switch1/1 -> out/1
  use_default/1 -> Switch1/2
  signal_out/1 -> Switch1/3
  in/1 -> signal_out/1

== system outp/OUTP/OUTP/VehHoldReq ==
  in : Inport
  use_default : Inport  Port=2
  KOUTP_VehHoldReq_flg_defval_C : Constant  Value=KOUTP_VehHoldReq_flg_defval
  KOUTP_VehHoldReq_flg_ovrdflg_C : Constant  Value=KOUTP_VehHoldReq_flg_ovrdflg
  KOUTP_VehHoldReq_flg_ovrdval_C : Constant  Value=KOUTP_VehHoldReq_flg_ovrdval
  KOUTP_VehHoldReq_flg_srvcflg_C : Constant  Value=KOUTP_VehHoldReq_flg_srvcflg
  KOUTP_VehHoldReq_flg_srvcval_C : Constant  Value=KOUTP_VehHoldReq_flg_srvcval
  Switch1 : Switch  Criteria=u2 ~= 0  Threshold=0.5
  signal_out : outp/signal_out
  out : Outport
  wires:
  in/1 -> signal_out/1
  signal_out/1 -> Switch1/3
  use_default/1 -> Switch1/2
  Switch1/1 -> out/1
  KOUTP_VehHoldReq_flg_srvcflg_C/1 -> signal_out/2
  KOUTP_VehHoldReq_flg_srvcval_C/1 -> signal_out/3
  KOUTP_VehHoldReq_flg_ovrdflg_C/1 -> signal_out/4
  KOUTP_VehHoldReq_flg_ovrdval_C/1 -> signal_out/5
  KOUTP_VehHoldReq_flg_defval_C/1 -> Switch1/1

== system outp/OUTP/OUTP/VehSpdLim ==
  in : Inport
  use_default : Inport  Port=2
  KOUTP_VehSpdLim_kph_defval_C : Constant  Value=KOUTP_VehSpdLim_kph_defval
  KOUTP_VehSpdLim_kph_ovrdflg_C : Constant  Value=KOUTP_VehSpdLim_kph_ovrdflg
  KOUTP_VehSpdLim_kph_ovrdval_C : Constant  Value=KOUTP_VehSpdLim_kph_ovrdval
  KOUTP_VehSpdLim_kph_srvcflg_C : Constant  Value=KOUTP_VehSpdLim_kph_srvcflg
  KOUTP_VehSpdLim_kph_srvcval_C : Constant  Value=KOUTP_VehSpdLim_kph_srvcval
  Switch1 : Switch  Criteria=u2 ~= 0  Threshold=0.5
  signal_out : outp/signal_out
  out : Outport
  wires:
  KOUTP_VehSpdLim_kph_defval_C/1 -> Switch1/1
  KOUTP_VehSpdLim_kph_ovrdval_C/1 -> signal_out/5
  KOUTP_VehSpdLim_kph_ovrdflg_C/1 -> signal_out/4
  KOUTP_VehSpdLim_kph_srvcval_C/1 -> signal_out/3
  KOUTP_VehSpdLim_kph_srvcflg_C/1 -> signal_out/2
  Switch1/1 -> out/1
  use_default/1 -> Switch1/2
  signal_out/1 -> Switch1/3
  in/1 -> signal_out/1

== system outp/OUTP/OUTP/VehSpdLimAppl ==
  in : Inport
  use_default : Inport  Port=2
  KOUTP_VehSpdLimAppl_flg_defval_C : Constant  Value=KOUTP_VehSpdLimAppl_flg_defval
  KOUTP_VehSpdLimAppl_flg_ovrdflg_C : Constant  Value=KOUTP_VehSpdLimAppl_flg_ovrdflg
  KOUTP_VehSpdLimAppl_flg_ovrdval_C : Constant  Value=KOUTP_VehSpdLimAppl_flg_ovrdval
  KOUTP_VehSpdLimAppl_flg_srvcflg_C : Constant  Value=KOUTP_VehSpdLimAppl_flg_srvcflg
  KOUTP_VehSpdLimAppl_flg_srvcval_C : Constant  Value=KOUTP_VehSpdLimAppl_flg_srvcval
  Switch1 : Switch  Criteria=u2 ~= 0  Threshold=0.5
  signal_out : outp/signal_out
  out : Outport
  wires:
  in/1 -> signal_out/1
  signal_out/1 -> Switch1/3
  use_default/1 -> Switch1/2
  Switch1/1 -> out/1
  KOUTP_VehSpdLimAppl_flg_srvcflg_C/1 -> signal_out/2
  KOUTP_VehSpdLimAppl_flg_srvcval_C/1 -> signal_out/3
  KOUTP_VehSpdLimAppl_flg_ovrdflg_C/1 -> signal_out/4
  KOUTP_VehSpdLimAppl_flg_ovrdval_C/1 -> signal_out/5
  KOUTP_VehSpdLimAppl_flg_defval_C/1 -> Switch1/1

== system outp/OUTP/OUTP/VirtualGearRatio ==
  in : Inport
  use_default : Inport  Port=2
  KOUTP_VirtualGearRatio_enum_defval_C : Constant  Value=KOUTP_VirtualGearRatio_enum_defval
  KOUTP_VirtualGearRatio_enum_ovrdflg_C : Constant  Value=KOUTP_VirtualGearRatio_enum_ovrdflg
  KOUTP_VirtualGearRatio_enum_ovrdval_C : Constant  Value=KOUTP_VirtualGearRatio_enum_ovrdval
  KOUTP_VirtualGearRatio_enum_srvcflg_C : Constant  Value=KOUTP_VirtualGearRatio_enum_srvcflg
  KOUTP_VirtualGearRatio_enum_srvcval_C : Constant  Value=KOUTP_VirtualGearRatio_enum_srvcval
  Switch1 : Switch  Criteria=u2 ~= 0  Threshold=0.5
  signal_out : outp/signal_out
  out : Outport
  wires:
  KOUTP_VirtualGearRatio_enum_defval_C/1 -> Switch1/1
  KOUTP_VirtualGearRatio_enum_ovrdval_C/1 -> signal_out/5
  KOUTP_VirtualGearRatio_enum_ovrdflg_C/1 -> signal_out/4
  KOUTP_VirtualGearRatio_enum_srvcval_C/1 -> signal_out/3
  KOUTP_VirtualGearRatio_enum_srvcflg_C/1 -> signal_out/2
  Switch1/1 -> out/1
  use_default/1 -> Switch1/2
  signal_out/1 -> Switch1/3
  in/1 -> signal_out/1

== stateflow chart OUTP/OUTP/Function Call Generator ADAS2 ==
  (default) -> (junction 7)
  (junction 7) -> (junction 8) [order 1] : [SampleTime_S<=C_TICK_TIME_S]
  (junction 7) -> (junction 9) [order 2] : {Timer=Timer+C_TICK_TIME_S;}
  (junction 8) -> (junction 11) : {FunCall;}
  (junction 9) -> (junction 10) [order 1] : [Timer>=SampleTime_S-0.0001]
  (junction 9) -> (junction 13) [order 2]
  (junction 10) -> (junction 12) : {FunCall;}
  (junction 11) -> (junction 15) : {Timer=0;}
  (junction 12) -> (junction 14) : {Timer=0;}
  (junction 14) -> (junction 13)
  (junction 15) -> (junction 14)
  data: SampleTime_S input double; C_TICK_TIME_S parameter double; Timer local single
  events: FunCall output FUNCTION_CALL_EVENT

== stateflow chart OUTP/OUTP/Function Call Generator ADAS3 ==
  (default) -> (junction 33)
  (junction 33) -> (junction 34) [order 1] : [SampleTime_S<=C_TICK_TIME_S]
  (junction 33) -> (junction 35) [order 2] : {Timer=Timer+C_TICK_TIME_S;}
  (junction 34) -> (junction 37) : {FunCall;}
  (junction 35) -> (junction 36) [order 1] : [Timer>=SampleTime_S-0.0001]
  (junction 35) -> (junction 39) [order 2]
  (junction 36) -> (junction 38) : {FunCall;}
  (junction 37) -> (junction 41) : {Timer=0;}
  (junction 38) -> (junction 40) : {Timer=0;}
  (junction 40) -> (junction 39)
  (junction 41) -> (junction 40)
  data: SampleTime_S input double; C_TICK_TIME_S parameter double; Timer local single
  events: FunCall output FUNCTION_CALL_EVENT

== stateflow chart OUTP/OUTP/Function Call Generator ADAS1 ==
  (default) -> (junction 59)
  (junction 59) -> (junction 60) [order 1] : [SampleTime_S<=C_TICK_TIME_S]
  (junction 59) -> (junction 61) [order 2] : {Timer=Timer+C_TICK_TIME_S;}
  (junction 60) -> (junction 63) : {FunCall;}
  (junction 61) -> (junction 62) [order 1] : [Timer>=SampleTime_S-0.0001]
  (junction 61) -> (junction 65) [order 2]
  (junction 62) -> (junction 64) : {FunCall;}
  (junction 63) -> (junction 67) : {Timer=0;}
  (junction 64) -> (junction 66) : {Timer=0;}
  (junction 66) -> (junction 65)
  (junction 67) -> (junction 66)
  data: SampleTime_S input double; C_TICK_TIME_S parameter double; Timer local single
  events: FunCall output FUNCTION_CALL_EVENT
